simulink model "GMCLIB_Clark_BAM_F16"  (Simulink 7.3)
settings: Solver=ode45  StartTime=0.0  StopTime=10.0  RelTol=1e-3
settings Model: Creator=B17364  LastModifiedBy=B17364

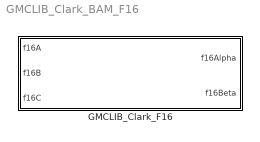
== system GMCLIB_Clark_BAM_F16 ==
  GMCLIB_Clark_F16 : Subsystem  mask(GMCLIB_Clark_F16){}
      mask help: Bit accurate model of Clarke transformation 3ph -> 2ph.
      mask init:
      | pos = get_param(gcb, 'Position');width = pos(3) - pos(1); height = pos(4) - pos(2);tX=width/2;tY=height*0.9;
      mask Display: color('black');port_label('input',1,'f16A');port_label('input',2,'f16B');port_label('input',3,'f16C');port_label('output',1,'f16Alpha');port_label('output',2,'f16Beta');color('black');disp('GMCLIB_Clark_F16');color('blue');text(tX,tY, 'BAM', 'horizontalAlignment', 'center');

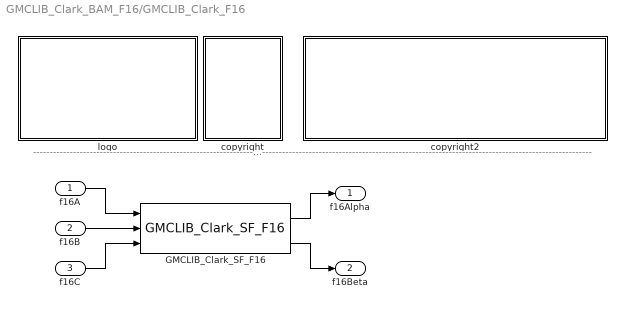
== system GMCLIB_Clark_BAM_F16/GMCLIB_Clark_F16 ==
  note: ---------------------------------------------------------------------------------------------------------------------------------------------------------------------------------------------------
  f16A : Inport  OutDataType=fixdt(1, 16)  OutScaling=2^0
  f16B : Inport  Port=2  OutDataType=fixdt(1, 16)  OutScaling=2^0
  f16C : Inport  Port=3  OutDataType=fixdt(1, 16)  OutScaling=2^0
  GMCLIB_Clark_SF_F16 : S-Function  FunctionName=GMCLIB_Clark_SF_F16  EnableBusSupport=off
  copyright : Subsystem
      mask Display: text(10,90,'FILE:');text(10,75,'DESRIPTION:')text(10,60,'COPYRIGHT:')text(10,45,'VERSION:')text(10,30,'DATE:')
  copyright2 : Subsystem
      mask Display: text(10,90,'GMCLIB_Clark_BAM_F16.mdl');text(10,75,'Clarke transformation.');text(10,60,'Freescale')text(10,45,'0.1');text(10,30,'29-Aug-2011');
  logo : Subsystem
      mask Display: image(imread('logo.jpg'))
  f16Alpha : Outport  OutDataType=fixdt(1, 16)  OutScaling=2^0
  f16Beta : Outport  Port=2  OutDataType=fixdt(1, 16)  OutScaling=2^0
  wires:
  f16A/1 -> GMCLIB_Clark_SF_F16/1
  f16B/1 -> GMCLIB_Clark_SF_F16/2
  f16C/1 -> GMCLIB_Clark_SF_F16/3
  GMCLIB_Clark_SF_F16/1 -> f16Alpha/1
  GMCLIB_Clark_SF_F16/2 -> f16Beta/1

== system GMCLIB_Clark_BAM_F16/GMCLIB_Clark_F16/copyright ==

== system GMCLIB_Clark_BAM_F16/GMCLIB_Clark_F16/copyright2 ==

== system GMCLIB_Clark_BAM_F16/GMCLIB_Clark_F16/logo ==
